simulink model "separator_test"  (R2019a)
settings: Solver=VariableStepAuto  StartTime=0.0  StopTime=100  RelTol=1e-3
libraries: simulink x1
settings Model: Creator=amah2  LastModifiedBy=kovim

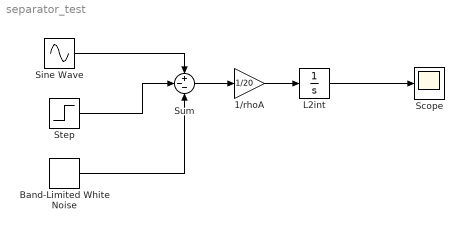
== system separator_test ==
  "1/rhoA " : Gain  Gain=1/20
  Band-Limited White Noise : simulink/Sources/Band-Limited White Noise  Cov=[0.1]  Ts=0.1  seed=[23341]
  "L2int " : Integrator  InitialCondition=1.0
  Scope : Scope
  Sine Wave : Sin  SampleTime=0
  Step : Step  SampleTime=0
  Sum : Sum  Inputs=+--
  wires:
  Sine Wave/1 -> Sum/1
  Step/1 -> Sum/2
  Band-Limited White Noise/1 -> Sum/3
  Sum/1 -> "1/rhoA "/1
  "1/rhoA "/1 -> "L2int "/1
  "L2int "/1 -> Scope/1
